simulink model "new_t_type_three_level"  (R2025b)
settings: Solver=ode4  StartTime=0.0  StopTime=0.2  FixedStep=1e-5  RelTol=1e-3  EnableMultiTasking=on
values from neighbouring files (symbols this model uses):
  tFault = 0.10    (= 0.1)    [collect_data_paper.m]    (also in diagnose_live.m; latency_sweep.m = tFaultAll(b); make_fig5.m = 0.105)
libraries: spsIGBTDiodeLib x12, spsVoltageMeasurementLib x4, spsCurrentMeasurementLib x3, spsNeutralLib x2, spsSeriesRLCBranchLib x2, simulink x2, spsThreePhaseSeriesRLCLoadLib x1, spsDCVoltageSourceLib x1, spspowerguiLib x1
settings Model: Creator=PEARL-SAAD  LastModifiedBy=rashe
settings SolverCC: AlgebraicLoopSolver=TrustRegion  AutoInsertRateTranBlk=on
settings DataIOCC: LimitDataPoints=on  SaveFormat=Array
settings OptimizationCC: ReuseModelBlockBuffer=off  LifeSpan=inf
settings DebuggingCC: SolverPrmCheckMsg=warning  UnconnectedInputMsg=warning  UnconnectedOutputMsg=warning  UnconnectedLineMsg=warning  SFUnexpectedBacktrackingDiag=warning  SFNoUnconditionalDefaultTransitionDiag=warning  SFExecutionAtInitializationDiag=none  ArithmeticOperatorsInVariantConditions=warning
settings HardwareCC: ProdBitPerPointer=32.0  ProdBitPerSizeT=32.0  ProdBitPerPtrDiffT=32.0  ProdLargestAtomicFloat=None  ProdIntDivRoundTo=Undefined  ProdEndianess=Unspecified  ProdWordSize=32.0  ProdHWDeviceType=32-bit Generic
settings ModelReferenceCC: EnableRefExpFcnMdlSchedulingChecks=on  PropagateSignalLabelsOutOfModel=off
settings SFSimCC: SimUseLocalCustomCode=off  CustomCodeUndefinedFunction=UseInterfaceOnly
settings RTWCC: RTWUseLocalCustomCode=off  GPUComputeCapability=3.5  DLArmComputeVersion=19.05
settings CodeAppCC: StateflowObjectComments=on
settings GRTTargetCC: TargetLangStandard=C89/C90 (ANSI)
settings ConfigComp: CovMetricSettings=dw  CovSaveCumulativeToWorkspaceVar=on  CovSaveSingleToWorkspaceVar=on  CovExternalEMLEnable=off  CovSFcnEnable=off
settings SimscapeCC: SimscapeNormalizeSystem=off

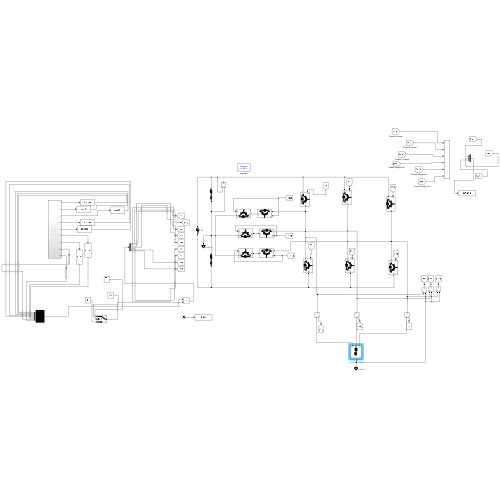
[thumbnail: Simulink's stored preview of the top-level diagram]
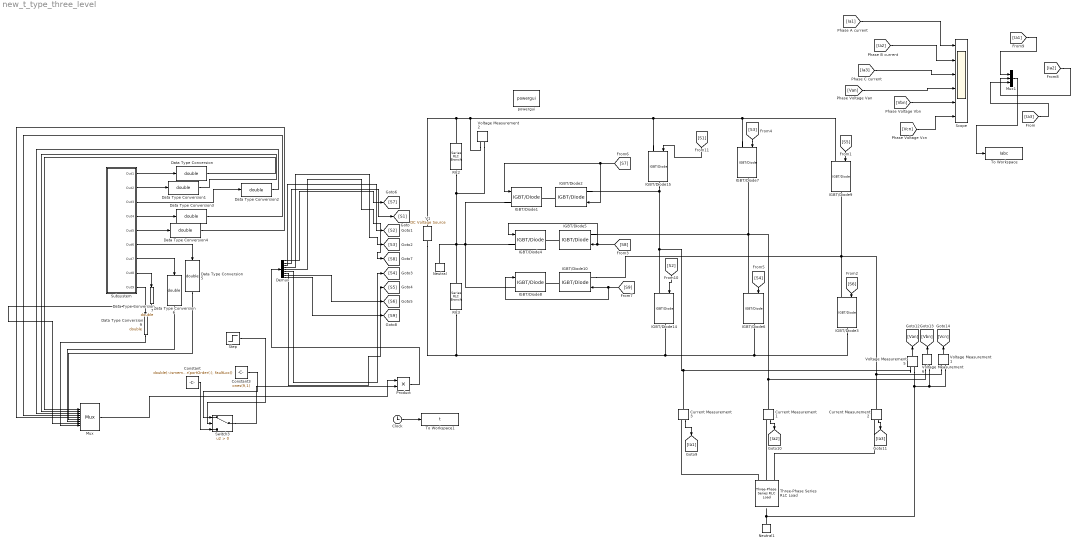
== system new_t_type_three_level ==
  Clock : Clock
  Constant : Constant  Value=double(~ismember(portOrder(:), faultLoc))
  Constant3 : Constant  Value=ones(9,1)
  Current Measurement1 : spsCurrentMeasurementLib/Current Measurement  PhasorSimulation=off  OutputType=Complex  PSBequivalent=0
  Current Measurement2 : spsCurrentMeasurementLib/Current Measurement  PhasorSimulation=off  OutputType=Complex  PSBequivalent=0
  Current Measurement3 : spsCurrentMeasurementLib/Current Measurement  PhasorSimulation=off  OutputType=Complex  PSBequivalent=0
  Data Type Conversion{,1..7,9} (9 alike) : DataTypeConversion  OutDataTypeStr=double  SaturateOnIntegerOverflow=off  RndMeth=Floor
  Demux : Demux  Outputs=9
  IGBT/Diode{1..10,14..15} (12 alike) : spsIGBTDiodeLib/IGBT//Diode  Ron=1e-3  Rs=1e5  Cs=inf  Measurements=off
  Mux : Mux  Inputs=9
  Mux1 : Mux  Inputs=3
  Neutral : spsNeutralLib/Neutral  LConnTagsString=a  NodeNumber=10
      settings: AttributesFormatString=node %<NodeNumber>  LibrarySourceBlock=sps_lib/Utilities/Neutral
  Neutral1 : spsNeutralLib/Neutral  LConnTagsString=a  NodeNumber=10
      settings: AttributesFormatString=node %<NodeNumber>  LibrarySourceBlock=sps_lib/Utilities/Neutral
  Product : Product
  RC2 : spsSeriesRLCBranchLib/Series RLC Branch  LConnTagsString=__new0  RConnTagsString=__new0  BranchType=RC  Resistance=.1  Inductance=1e-3  SetiL0=off  InitialCurrent=0  Capacitance=4.7e-3  Setx0=off  InitialVoltage=0  Measurements=None
  RC3 : spsSeriesRLCBranchLib/Series RLC Branch  LConnTagsString=__new0  RConnTagsString=__new0  BranchType=RC  Resistance=.1  Inductance=1e-3  SetiL0=off  InitialCurrent=0  Capacitance=4.7e-3  Setx0=off  InitialVoltage=0  Measurements=None
  Scope : Scope  NumInputPorts=6
      settings: ActiveDisplayYMinimum=-113.95043374040463  ActiveDisplayYMaximum=113.77631340648257  DataLoggingVariableName=ttype
  Step : Step  Time=tFault  Before=1  After=0  SampleTime=0
  Subsystem : Subsystem
  Switch3 : Switch  Criteria=u2 > Threshold  SaturateOnIntegerOverflow=off  InputSameDT=off
  Three-Phase Series RLC Load : spsThreePhaseSeriesRLCLoadLib/Three-Phase Series RLC Load  LConnTagsString=A|B|C  Configuration=Y (floating)  NominalVoltage=555  Vabc=[1e3 1e3 1e3]  Vabcp=[1e3 1e3 1e3]  NominalFrequency=50  UnbalancedPower=off  ActivePower=Pload  InductivePower=Qload  CapacitivePower=0  Pabc=[10e3 9e3 11e3]  QLabc=[100 90 110]  QCabc=[100 90 110]  Pabcp=[10e3 9e3 11e3]  QLabcp=[100 90 110]  QCabcp=[100 90 110]  Measurements=None  LoadType=constant I
  To Workspace : ToWorkspace  VariableName=Iabc  SampleTime=1/25000
  To Workspace1 : ToWorkspace  VariableName=t  SaveFormat=Timeseries  SampleTime=-1
  V1 : spsDCVoltageSourceLib/DC Voltage Source  Amplitude=1000  Measurements=None
  Voltage Measurement{1..2,5..6} (4 alike) : spsVoltageMeasurementLib/Voltage Measurement  PhasorSimulation=off  OutputType=Complex  PSBequivalent=0
  powergui : spspowerguiLib/powergui  Priority=1  SimulationMode=Discrete  SampleTime=1e-5  frequency=60  Iterations=50  frequencyindice=0  Pbase=100e6  ErrMax=1e-4  UnitsV=kV  UnitsW=MW  buscounter=0  FunctionMessages=off  echomessages=off  EnableUseOfTLC=off  CurrentSourceSwitches=on  DisableSnubberDevices=off  DisableRonSwitches=off  DisableVfSwitches=off  DisplayEquations=off  AutomaticDiscreteSolvers=off  SolverType=Tustin  Interpol=off  ExternalGateDelay=off  methode=off  Ts=0  x0status=blocks  SPID=off  SwTol=0  HookPort=off  NonlinearTolerance=1e-4  nMaxIteration=100  ContinueOnMaxIteration=off  RestoreLinks=warning  ResistiveCurrentMeasurement=off  Frange=[0:2:500]  Ylog=off  Xlog=on  ShowGrid=off  save=off  variable=ZData  structure=nine_level_SHEPWM  ZoomFFT=off  StartTime=0.08  cycles=1  DisplayStyle=1  fundamental=50  FreqAxis=on  MaxFrequency=2500  frequencyindicesteady=1  RmsSteady=1  display=off
  wires:
  [S6] -> IGBT/Diode3/1
  [S8] -> IGBT/Diode4/1, IGBT/Diode5/1
  [S7] -> IGBT/Diode1/1, IGBT/Diode2/1
  [S3] -> IGBT/Diode7/1
  [S4] -> IGBT/Diode6/1
  [S5] -> IGBT/Diode9/1
  [S9] -> IGBT/Diode8/1, IGBT/Diode10/1
  Current Measurement3/1 -> [Ia1]
  Current Measurement1/1 -> [Ia2]
  Current Measurement2/1 -> [Ia3]
  Voltage Measurement5/1 -> [Van]
  Voltage Measurement6/1 -> [Vbn]
  Voltage Measurement1/1 -> [Vcn]
  [Van] -> Scope/4
  [Vbn] -> Scope/5
  [Vcn] -> Scope/6
  [Ia1] -> Scope/1
  [Ia2] -> Scope/2
  [Ia3] -> Scope/3
  Clock/1 -> To Workspace1/1
  [S1] -> IGBT/Diode15/1
  [S2] -> IGBT/Diode14/1
  Mux/1 -> Product/1
  Switch3/1 -> Product/2
  Constant3/1 -> Switch3/1
  Step/1 -> Switch3/2
  Constant/1 -> Switch3/3
  Product/1 -> Demux/1
  Subsystem/1(Out1) -> Data Type Conversion/1
  Subsystem/9(Out9) -> Data Type Conversion9/1
  Subsystem/8(Out8) -> Data Type Conversion7/1
  Subsystem/2(Out2) -> Data Type Conversion1/1
  Subsystem/3(Out3) -> Data Type Conversion2/1
  Subsystem/4(Out4) -> Data Type Conversion3/1
  Subsystem/5(Out5) -> Data Type Conversion4/1
  Subsystem/6(Out6) -> Data Type Conversion5/1
  Subsystem/7(Out7) -> Data Type Conversion6/1
  Demux/1 -> [S7]
  Demux/2 -> [S1]
  Demux/3 -> [S2]
  Demux/4 -> [S3]
  Demux/5 -> [S8]
  Demux/6 -> [S4]
  Demux/7 -> [S5]
  Demux/8 -> [S6]
  Data Type Conversion/1 -> Mux/1
  Data Type Conversion1/1 -> Mux/2
  Data Type Conversion2/1 -> Mux/3
  Data Type Conversion3/1 -> Mux/4
  Data Type Conversion4/1 -> Mux/5
  Data Type Conversion5/1 -> Mux/6
  Data Type Conversion6/1 -> Mux/7
  Data Type Conversion7/1 -> Mux/8
  Data Type Conversion9/1 -> Mux/9
  Demux/9 -> [S9]
  [Ia1] -> Mux1/1
  [Ia2] -> Mux1/2
  [Ia3] -> Mux1/3
  Mux1/1 -> To Workspace/1
  connections:
  V1/RConn1 -- RC2/LConn1 -- Voltage Measurement2/LConn1 -- IGBT/Diode15/LConn1 -- IGBT/Diode7/LConn1 -- IGBT/Diode9/LConn1
  IGBT/Diode3/RConn1 -- IGBT/Diode6/RConn1 -- IGBT/Diode14/RConn1 -- RC3/RConn1 -- V1/LConn1
  RC2/RConn1 -- Voltage Measurement2/LConn2 -- Neutral/LConn1 -- IGBT/Diode8/LConn1 -- IGBT/Diode1/LConn1 -- IGBT/Diode4/LConn1 -- RC3/LConn1
  IGBT/Diode2/RConn1 -- IGBT/Diode1/RConn1
  IGBT/Diode5/RConn1 -- IGBT/Diode4/RConn1
  IGBT/Diode10/RConn1 -- IGBT/Diode8/RConn1
  Three-Phase Series RLC Load/LConn1 -- Current Measurement3/RConn1
  Three-Phase Series RLC Load/LConn2 -- Current Measurement1/RConn1
  Three-Phase Series RLC Load/LConn3 -- Current Measurement2/RConn1
  IGBT/Diode6/LConn1 -- Current Measurement1/LConn1 -- Voltage Measurement6/LConn1 -- IGBT/Diode5/LConn1 -- IGBT/Diode7/RConn1
  IGBT/Diode3/LConn1 -- Voltage Measurement1/LConn1 -- Current Measurement2/LConn1 -- IGBT/Diode10/LConn1 -- IGBT/Diode9/RConn1
  IGBT/Diode2/LConn1 -- Voltage Measurement5/LConn1 -- Current Measurement3/LConn1 -- IGBT/Diode14/LConn1 -- IGBT/Diode15/RConn1
  Neutral1/LConn1 -- Voltage Measurement1/LConn2 -- Voltage Measurement6/LConn2 -- Voltage Measurement5/LConn2

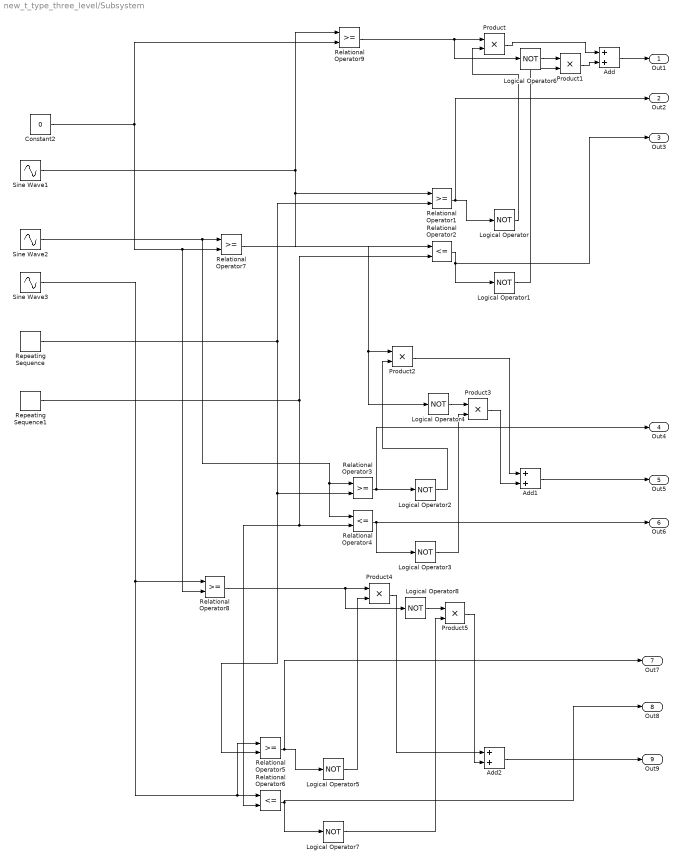
== system new_t_type_three_level/Subsystem ==
  Add : Sum
  Add1 : Sum
  Add2 : Sum
  Constant2 : Constant  Value=0
  Logical Operator{,1..8} (9 alike) : Logic  Operator=NOT  AllPortsSameDT=off  OutDataTypeStr=boolean
  Product{,1..5} (6 alike) : Product
  Relational Operator{1,3,5,7..9} (6 alike) : RelationalOperator  OutDataTypeStr=boolean  InputSameDT=off
  Relational Operator2 : RelationalOperator  Operator=<=  OutDataTypeStr=boolean  InputSameDT=off
  Relational Operator4 : RelationalOperator  Operator=<=  OutDataTypeStr=boolean  InputSameDT=off
  Relational Operator6 : RelationalOperator  Operator=<=  OutDataTypeStr=boolean  InputSameDT=off
  Repeating Sequence : simulink/Sources/Repeating Sequence  rep_seq_t=[0 0.5/5000 1/5000]  rep_seq_y=[0 1 0]
  Repeating Sequence1 : simulink/Sources/Repeating Sequence  rep_seq_t=[0 0.5/6000 1/6000]  rep_seq_y=[-1 0 -1]
  Sine Wave1 : Sin  Amplitude=.95  Frequency=100*pi  SampleTime=0
  Sine Wave2 : Sin  Amplitude=.95  Frequency=100*pi  Phase=2*pi/3  SampleTime=0
  Sine Wave3 : Sin  Amplitude=.95  Frequency=100*pi  Phase=4*pi/3  SampleTime=0
  Out1 : Outport
  Out2 : Outport  Port=2
  Out3 : Outport  Port=3
  Out4 : Outport  Port=4
  Out5 : Outport  Port=5
  Out6 : Outport  Port=6
  Out7 : Outport  Port=7
  Out8 : Outport  Port=8
  Out9 : Outport  Port=9
  wires:
  Logical Operator3/1 -> Product3/2
  Logical Operator1/1 -> Product1/2
  Product2/1 -> Add1/1
  Product1/1 -> Add/2
  Logical Operator5/1 -> Product4/2
  Add2/1 -> Out9/1
  Product3/1 -> Add1/2
  Logical Operator/1 -> Product/2
  Product4/1 -> Add2/1
  Logical Operator8/1 -> Product5/1
  Relational Operator6/1 -> Logical Operator7/1, Out8/1
  Logical Operator4/1 -> Product3/1
  Add1/1 -> Out5/1
  Product5/1 -> Add2/2
  Relational Operator1/1 -> Out2/1, Logical Operator/1
  Constant2/1 -> Relational Operator8/2, Relational Operator7/2, Relational Operator9/2
  Relational Operator8/1 -> Logical Operator8/1, Product4/1
  Logical Operator2/1 -> Product2/2
  Relational Operator3/1 -> Out4/1, Logical Operator2/1
  Repeating Sequence1/1 -> Relational Operator2/2, Relational Operator4/2, Relational Operator6/2
  Repeating Sequence/1 -> Relational Operator1/2, Relational Operator3/2, Relational Operator5/2
  Sine Wave3/1 -> Relational Operator5/1, Relational Operator6/1, Relational Operator8/1
  Relational Operator9/1 -> Logical Operator6/1, Product/1
  Product/1 -> Add/1
  Logical Operator7/1 -> Product5/2
  Sine Wave2/1 -> Relational Operator3/1, Relational Operator4/1, Relational Operator7/1
  Add/1 -> Out1/1
  Relational Operator2/1 -> Out3/1, Logical Operator1/1
  Relational Operator5/1 -> Out7/1, Logical Operator5/1
  Logical Operator6/1 -> Product1/1
  Relational Operator7/1 -> Logical Operator4/1, Product2/1
  Relational Operator4/1 -> Out6/1, Logical Operator3/1
  Sine Wave1/1 -> Relational Operator1/1, Relational Operator2/1, Relational Operator9/1
